simulink library "OpenFlightUtilLib"  (R2016b)
settings: Solver=VariableStepAuto  StartTime=0.0  StopTime=10.0  RelTol=1e-3
undefined symbols (not defined in the file or in its folder): SampleTime
libraries: OpenFlightUtilLib x46, simulink x7, dspmtrx3 x1
settings Model: Creator=UAVLAB  LastModifiedBy=rega0051

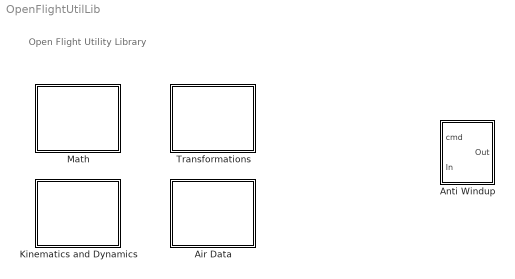
== system OpenFlightUtilLib ==
  note: Open Flight Utility Library
  Air Data : Subsystem
  Anti Windup : Subsystem  mask(Integrator Anti-Windup){MAX_DEF=0, MIN_DEF=0, gain_sign=off}
      mask prompts: MAX_DEF "Maximum surface deflection limit"; MIN_DEF "Minimum surface deflection limit"; gain_sign "Positive gains in control law"
      mask help:
      | This block uses boolean logic to eliminate integrator windup.
      | It compares the sign of the error between reference and output,
      | and the sign and position of the surface being controlled.
      mask Help:
      | See the "READ ME" block under the mask for a more thorough explanation of
      | how this block works.
  Kinematics and Dynamics : Subsystem
  Math : Subsystem
  Transformations : Subsystem

== system OpenFlightUtilLib/Air Data ==
  note: Air Data
  Angle_of_Attack : Subsystem  mask(Angle of Attack){}
      mask help: Compute the angle of attack from component velocities.
  Angle_of_Flank : Subsystem  mask(Angle of Flank){}
      mask help: Compute the angle of flank from component velocities.
  Angle_of_Sideslip : Subsystem  mask(Angle of Sideslip){}
      mask help: Compute the angle of sideslip from component velocities.
  ComponentVelocities : Subsystem  mask(Component Velocities){}
      mask help: Compute the component velocities from the True Airpeed, Angle of Attack, and Angle of Sideslip.
  ComponentVelocities_Flank : Subsystem  mask(Component Velocities){}
      mask help: Compute the component velocities from the True Airpeed, Angle of Attack, and Angle of Flank.
  DynamicPressure : Subsystem  mask(Dynamic Pressure){}
      mask help: Compute the Dynamic Pressure
  Mach : Subsystem  mask(Mach Number){}
      mask help: Compute the Mach Number
  True_Airspeed : Subsystem  mask(True Airspeed){}
      mask help: Compute the true airspeed from component velocities.
  WindAngles : Subsystem  mask(Wind Angles){}
      mask help: Compute the True Airpeed, Angle of Attack, and Angle of Sideslip from component velocities.
  WindAngles_Flank : Subsystem  mask(Wind Angles){}
      mask help: Compute the True Airpeed, Angle of Attack, and Angle of Flank from component velocities.

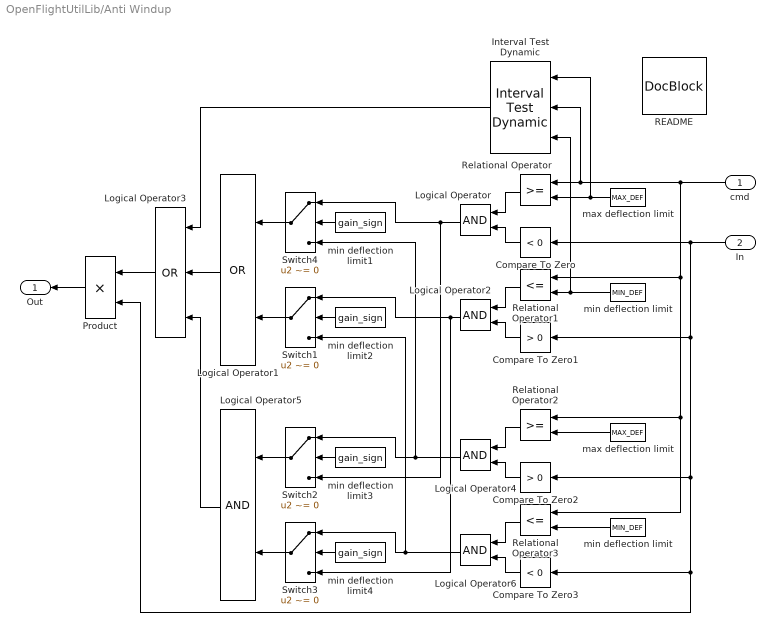
== system OpenFlightUtilLib/Anti Windup ==
  cmd : Inport
  In : Inport  Port=2
  Compare To Zero : simulink/Logic and Bit Operations/Compare To Zero  SystemSampleTime=-1  relop=<  LogicOutDataTypeMode=uint8
  Compare To Zero1 : simulink/Logic and Bit Operations/Compare To Zero  SystemSampleTime=-1  relop=>  LogicOutDataTypeMode=uint8
  Compare To Zero2 : simulink/Logic and Bit Operations/Compare To Zero  SystemSampleTime=-1  relop=>  LogicOutDataTypeMode=uint8
  Compare To Zero3 : simulink/Logic and Bit Operations/Compare To Zero  SystemSampleTime=-1  relop=<  LogicOutDataTypeMode=uint8
  Interval Test Dynamic : simulink/Logic and Bit Operations/Interval Test Dynamic  SystemSampleTime=-1  IntervalClosedRight=on  IntervalClosedLeft=on  LogicOutDataTypeMode=boolean
  Logical Operator{,2,4..6} (5 alike) : Logic  AllPortsSameDT=off  OutDataTypeStr=boolean  SampleTime=SampleTime
  Logical Operator1 : Logic  Operator=OR  AllPortsSameDT=off  OutDataTypeStr=boolean  SampleTime=SampleTime
  Logical Operator3 : Logic  Operator=OR  Inputs=3  AllPortsSameDT=off  OutDataTypeStr=boolean  SampleTime=SampleTime
  Product : Product  RndMeth=Zero
  README : simulink/Model-Wide Utilities/DocBlock  SystemSampleTime=-1  DocumentType=Text
      content=|
      | This block uses anti-windup logic to either stop or continue integrating.
      |
      | The first input signal, 'cmd', must come from the control surface command
      | that is the output of the controller. For instance, if the outputs of a PI
      | control phi tracker (with anti-windup) and a P control roll damper are
      | summed and sent to the aileron command, then the summed value must be fed
      | back into the 'cmd' input of this anti-windup block, as opposed to just the
      | output of the phi tracker.
      |
      | The second input signal, 'In', must come from the error that is being fed
      | into the control law.
      |
      | The output signal, 'Out' must feed into the error integrator block.
      |
      | For the anti-windup to work as intended, a saturation block must be placed
      | on the ouput of the control command being fed to the associated actuator.
      | If the controller is in delta coordinates, the limits in the saturation
      | block must be the actuator limits minus the trimmed control surface value.
      | For instance, for and aileron command, the limits would be:
      | Upper Limit: AC.Actuator.r_aileron.PosLim-TrimCondition.Inputs.r_aileron
      | Lower Limit: AC.Actuator.r_aileron.NegLim-TrimCondition.Inputs.r_aileron
      |
      | Depending on which surface is being controlled, the windup logic may
      | change. The default logic for this block is the following:
      |
      | For input u, saturation limits Umax and Umin, and error e,
      | If u is in bounds, do nothing
      | If u >= Umax AND e < 0, stop integrating
      | If u >= Umax AND e > 0, continue integrating
      | If u <= Umin AND e < 0, continue integrating
      | If u <= Umin AND e > 0, stop integrating
      |
      | This is the logic for a plant transfer function with a negative gain. In
      | other words, a positive input gives a negative response, which is usually
      | the case with flight dynamics. If the plant transfer function does not have
      | a negative gain, the logic will need to be reversed. In this case, the
      | inequalities on the error logic must be switched, so
      | If u is in bounds, do nothing
      | If u >= Umax AND e > 0, stop integrating
      | If u >= Umax AND e < 0, continue integrating
      | If u <= Umin AND e > 0, continue integrating
      | If u <= Umin AND e < 0, stop integrating
  Relational Operator : RelationalOperator  OutDataTypeStr=boolean  RndMeth=Nearest
  Relational Operator1 : RelationalOperator  Operator=<=  OutDataTypeStr=boolean  RndMeth=Nearest
  Relational Operator2 : RelationalOperator  OutDataTypeStr=boolean  RndMeth=Nearest
  Relational Operator3 : RelationalOperator  Operator=<=  OutDataTypeStr=boolean  RndMeth=Nearest
  Switch{1..4} (4 alike) : Switch  Criteria=u2 ~= 0  SampleTime=SampleTime
  max deflection limit : Constant  Value=MAX_DEF  SampleTime=SampleTime
  "max deflection limit " : Constant  Value=MAX_DEF  SampleTime=SampleTime
  min deflection limit : Constant  Value=MIN_DEF  SampleTime=SampleTime
  "min deflection limit " : Constant  Value=MIN_DEF  SampleTime=SampleTime
  min deflection limit{1..4} (4 alike) : Constant  Value=gain_sign  SampleTime=SampleTime
  Out : Outport
  wires:
  Logical Operator5/1 -> Logical Operator3/3
  "max deflection limit "/1 -> Relational Operator2/2
  "min deflection limit "/1 -> Relational Operator3/2
  Relational Operator3/1 -> Logical Operator6/1
  Compare To Zero3/1 -> Logical Operator6/2
  Relational Operator2/1 -> Logical Operator4/1
  Compare To Zero2/1 -> Logical Operator4/2
  Interval Test Dynamic/1 -> Logical Operator3/1
  Logical Operator1/1 -> Logical Operator3/2
  Logical Operator3/1 -> Product/1
  Product/1 -> Out/1
  min deflection limit/1 -> Interval Test Dynamic/3, Relational Operator1/2
  Relational Operator1/1 -> Logical Operator2/1
  Compare To Zero1/1 -> Logical Operator2/2
  In/1 -> Product/2, Compare To Zero3/1, Compare To Zero2/1, Compare To Zero1/1, Compare To Zero/1
  Relational Operator/1 -> Logical Operator/1
  Compare To Zero/1 -> Logical Operator/2
  cmd/1 -> Relational Operator3/1, Relational Operator2/1, Relational Operator1/1, Interval Test Dynamic/2, Relational Operator/1
  max deflection limit/1 -> Interval Test Dynamic/1, Relational Operator/2
  min deflection limit2/1 -> Switch1/2
  min deflection limit3/1 -> Switch2/2
  min deflection limit4/1 -> Switch3/2
  Switch2/1 -> Logical Operator5/1
  Switch3/1 -> Logical Operator5/2
  Switch1/1 -> Logical Operator1/2
  Switch4/1 -> Logical Operator1/1
  min deflection limit1/1 -> Switch4/2
  Logical Operator/1 -> Switch4/1, Switch2/3
  Logical Operator2/1 -> Switch1/1, Switch3/3
  Logical Operator4/1 -> Switch2/1, Switch4/3
  Logical Operator6/1 -> Switch3/1, Switch1/3

== system OpenFlightUtilLib/Kinematics and Dynamics ==
  note: Kinematics and Dynamics
  AngMomentum : Subsystem
  AngMomentumInv : Subsystem
  RelAccel : Subsystem
  RelAccelRigid : Subsystem
  RelForce : Subsystem
  RelForceRigid : Subsystem
  RelVel : Subsystem
  RelVelRigid : Subsystem
  TransMomentum : Subsystem
  TransMomentumInv : Subsystem

== system OpenFlightUtilLib/Math ==
  note: Simple Math
  CrossProduct3 : Subsystem  mask(Corss Product (3x3)){}
      mask help: Computes the cross product of two vectors of length 3.
  NormFrobenious : Subsystem
  NormL2 : Subsystem  mask(Norm L2){}
      mask help:
      | Computes the L2 Norm of a vector.
      | y = sqrt(x1^2 + x2^2 + ... + xn^2)
      mask Display: disp('||u||2');
  Psi_180_2_360 : Subsystem
  SkewSymmetric3 : Subsystem  mask(Skew Symmetric (3x3)){}
      mask help:
      | Compute the skew symmetric matrix of a vector of length 3.
      | M = [0, -V(3), V(2); V(3), 0, -V(1); -V(2), V(1), 0]
  ZeroProtect : Subsystem  mask(Zero Protection){epsilon=eps}
      mask prompts: epsilon "Epsilon value:"
      mask help:
      | Protection for divide by zero.
      | out = sign(in) * max(abs(in), eps)

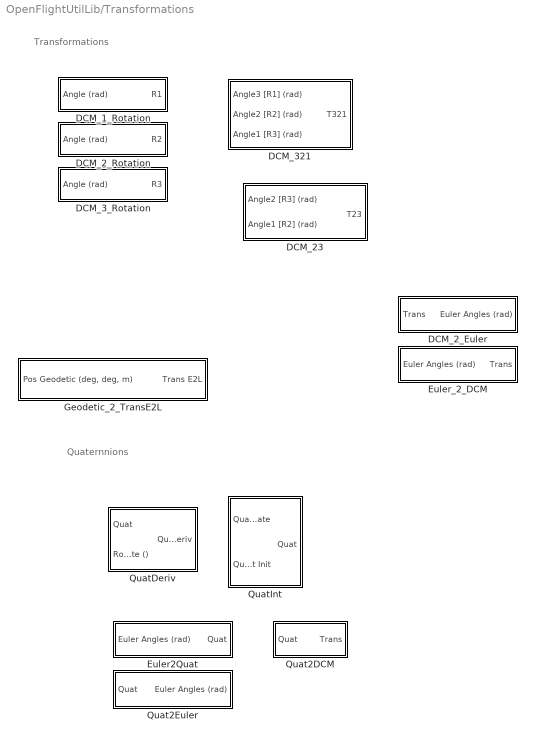
== system OpenFlightUtilLib/Transformations ==
  note: Quaternnions
  note: Transformations
  DCM_1_Rotation : Subsystem
  DCM_23 : Subsystem
  DCM_2_Euler : Subsystem
  DCM_2_Rotation : Subsystem
  DCM_321 : Subsystem
  DCM_3_Rotation : Subsystem
  Euler2Quat : Subsystem
  Euler_2_DCM : Subsystem
  Geodetic_2_TransE2L : Subsystem
  Quat2DCM : Subsystem
  Quat2Euler : Subsystem
  QuatDeriv : Subsystem
  QuatInt : Subsystem

== system OpenFlightUtilLib/Air Data/Angle_of_Attack ==
  note: alpha = atan(w / u)
  note: Convert Velocity Components to Angles of Attack
  u : Inport
  w : Inport  Port=2
  Trigonometric Function : Trigonometry  Operator=atan2
  alpha (rad) : Outport
  wires:
  Trigonometric Function/1 -> alpha (rad)/1
  u/1 -> Trigonometric Function/2
  w/1 -> Trigonometric Function/1

== system OpenFlightUtilLib/Air Data/Angle_of_Flank ==
  note: Convert Velocity Components to Angles of Flank
  note: flank = atan(v / u)
  u : Inport
  v : Inport  Port=2
  Trigonometric Function1 : Trigonometry  Operator=atan2
  flank (rad) : Outport
  wires:
  Trigonometric Function1/1 -> flank (rad)/1
  v/1 -> Trigonometric Function1/1
  u/1 -> Trigonometric Function1/2

== system OpenFlightUtilLib/Air Data/Angle_of_Sideslip ==
  note: beta = asin(v / V)
  note: Convert Velocity Components to Angles of Sideslip
  vTrue : Inport
  v : Inport  Port=2
  Product2 : Product  Inputs=*/  RndMeth=Zero
  Trigonometric Function1 : Trigonometry  Operator=asin
  ZeroProtect : OpenFlightUtilLib/Math/ZeroProtect  epsilon=eps
  beta (rad) : Outport
  wires:
  ZeroProtect/1 -> Product2/2
  Trigonometric Function1/1 -> beta (rad)/1
  Product2/1 -> Trigonometric Function1/1
  v/1 -> Product2/1
  vTrue/1 -> ZeroProtect/1

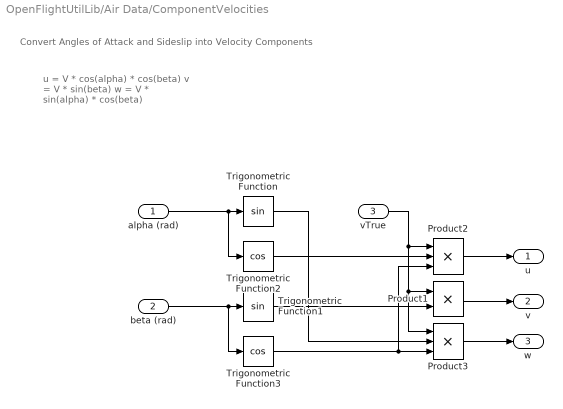
== system OpenFlightUtilLib/Air Data/ComponentVelocities ==
  note: u = V * cos(alpha) * cos(beta)
      | v = V * sin(beta)
      | w = V * sin(alpha) * cos(beta)
  note: Convert Angles of Attack and Sideslip into Velocity Components
  alpha (rad) : Inport
  beta (rad) : Inport  Port=2
  vTrue : Inport  Port=3
  Product1 : Product  Inputs=**  RndMeth=Zero
  Product2 : Product  Inputs=***  RndMeth=Zero
  Product3 : Product  Inputs=***  RndMeth=Zero
  Trigonometric Function : Trigonometry
  Trigonometric Function1 : Trigonometry
  Trigonometric Function2 : Trigonometry  Operator=cos
  Trigonometric Function3 : Trigonometry  Operator=cos
  u : Outport
  v : Outport  Port=2
  w : Outport  Port=3
  wires:
  Product3/1 -> w/1
  Product1/1 -> v/1
  beta (rad)/1 -> Trigonometric Function1/1, Trigonometric Function3/1
  alpha (rad)/1 -> Trigonometric Function/1, Trigonometric Function2/1
  Product2/1 -> u/1
  Trigonometric Function1/1 -> Product1/2
  Trigonometric Function/1 -> Product3/2
  vTrue/1 -> Product2/1, Product1/1, Product3/1
  Trigonometric Function2/1 -> Product2/2
  Trigonometric Function3/1 -> Product2/3, Product3/3

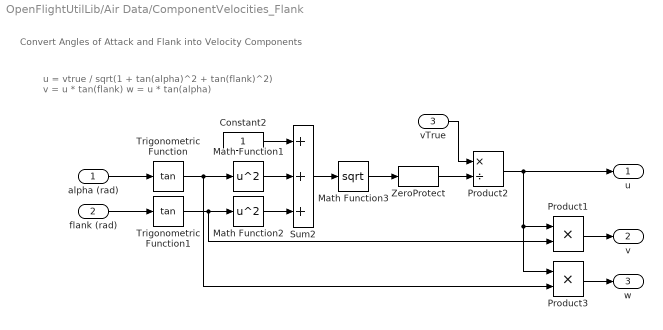
== system OpenFlightUtilLib/Air Data/ComponentVelocities_Flank ==
  note: Convert Angles of Attack and Flank into Velocity Components
  note: u = vtrue / sqrt(1 + tan(alpha)^2 + tan(flank)^2)
      | v = u * tan(flank)
      | w = u * tan(alpha)
  alpha (rad) : Inport
  flank (rad) : Inport  Port=2
  vTrue : Inport  Port=3
  Constant2 : Constant
  Math Function1 : Math  Operator=square  SaturateOnIntegerOverflow=on
  Math Function2 : Math  Operator=square  SaturateOnIntegerOverflow=on
  Math Function3 : Math  Operator=sqrt  SaturateOnIntegerOverflow=on
  Product1 : Product  Inputs=**  RndMeth=Zero
  Product2 : Product  Inputs=*/  RndMeth=Zero
  Product3 : Product  Inputs=**  RndMeth=Zero
  Sum2 : Sum  Inputs=+++
  Trigonometric Function : Trigonometry  Operator=tan
  Trigonometric Function1 : Trigonometry  Operator=tan
  ZeroProtect : OpenFlightUtilLib/Math/ZeroProtect  epsilon=eps
  u : Outport
  v : Outport  Port=2
  w : Outport  Port=3
  wires:
  vTrue/1 -> Product2/1
  Sum2/1 -> Math Function3/1
  Math Function3/1 -> ZeroProtect/1
  Trigonometric Function/1 -> Math Function1/1, Product3/2
  Trigonometric Function1/1 -> Math Function2/1, Product1/2
  Product2/1 -> u/1, Product1/1, Product3/1
  alpha (rad)/1 -> Trigonometric Function/1
  flank (rad)/1 -> Trigonometric Function1/1
  Product1/1 -> v/1
  Product3/1 -> w/1
  Constant2/1 -> Sum2/1
  Math Function1/1 -> Sum2/2
  Math Function2/1 -> Sum2/3
  ZeroProtect/1 -> Product2/2

== system OpenFlightUtilLib/Air Data/DynamicPressure ==
  note: qBar = 0.5 * rho * V^2
  note: Compute Dynamic Pressure
  vTrue : Inport
  density : Inport  Port=2
  Gain : Gain  Gain=1/2
  Math Function : Math  Operator=square  SaturateOnIntegerOverflow=on
  Product2 : Product  Inputs=**  RndMeth=Zero
  qBar : Outport
  wires:
  density/1 -> Product2/2
  vTrue/1 -> Math Function/1
  Product2/1 -> Gain/1
  Gain/1 -> qBar/1
  Math Function/1 -> Product2/1

== system OpenFlightUtilLib/Air Data/Mach ==
  note: Compute Mach Number
  note: mach = vTrue / vSound
  vTrue : Inport
  vSound : Inport  Port=2
  Product2 : Product  Inputs=*/  RndMeth=Zero
  ZeroProtect : OpenFlightUtilLib/Math/ZeroProtect  epsilon=eps
  mach : Outport
  wires:
  Product2/1 -> mach/1
  vSound/1 -> ZeroProtect/1
  vTrue/1 -> Product2/1
  ZeroProtect/1 -> Product2/2

== system OpenFlightUtilLib/Air Data/True_Airspeed ==
  note: V = sqrt(u^2 + v^2 + w^2)
  note: Convert Velocity Components to True Airspeed
  u : Inport
  v : Inport  Port=2
  w : Inport  Port=3
  Mux : Mux  Inputs=3
  NormL2 : OpenFlightUtilLib/Math/NormL2
  vTrue : Outport
  wires:
  Mux/1 -> NormL2/1
  u/1 -> Mux/1
  v/1 -> Mux/2
  w/1 -> Mux/3
  NormL2/1 -> vTrue/1

== system OpenFlightUtilLib/Air Data/WindAngles ==
  note: Convert Velocity Components to True Airspeed, Angles of Attack, and Sideslip
  u : Inport
  v : Inport  Port=2
  w : Inport  Port=3
  Angle_of_Attack : OpenFlightUtilLib/Air Data/Angle_of_Attack
  Angle_of_Sideslip1 : OpenFlightUtilLib/Air Data/Angle_of_Sideslip
  True_Airspeed : OpenFlightUtilLib/Air Data/True_Airspeed
  vTrue : Outport
  alpha (rad) : Outport  Port=2
  beta (rad) : Outport  Port=3
  wires:
  True_Airspeed/1 -> Angle_of_Sideslip1/1, vTrue/1
  Angle_of_Attack/1 -> alpha (rad)/1
  Angle_of_Sideslip1/1 -> beta (rad)/1
  u/1 -> True_Airspeed/1, Angle_of_Attack/1
  v/1 -> True_Airspeed/2, Angle_of_Sideslip1/2
  w/1 -> True_Airspeed/3, Angle_of_Attack/2

== system OpenFlightUtilLib/Air Data/WindAngles_Flank ==
  note: V = sqrt(u^2 + v^2 + w^2)
      | alpha = atan(w / u)
      | flank = atan(v / u)
  note: Convert Velocity Components to Angles of Attack and Flank
  u : Inport
  v : Inport  Port=2
  w : Inport  Port=3
  Angle_of_Attack : OpenFlightUtilLib/Air Data/Angle_of_Attack
  Angle_of_Flank : OpenFlightUtilLib/Air Data/Angle_of_Flank
  True_Airspeed : OpenFlightUtilLib/Air Data/True_Airspeed
  vTrue : Outport
  alpha (rad) : Outport  Port=2
  flank (rad) : Outport  Port=3
  wires:
  u/1 -> True_Airspeed/1, Angle_of_Flank/1, Angle_of_Attack/1
  v/1 -> Angle_of_Flank/2, True_Airspeed/2
  w/1 -> Angle_of_Attack/2, True_Airspeed/3
  True_Airspeed/1 -> vTrue/1
  Angle_of_Attack/1 -> alpha (rad)/1
  Angle_of_Flank/1 -> flank (rad)/1

== system OpenFlightUtilLib/Kinematics and Dynamics/AngMomentum ==
  note: Rigid Body Conservation of Angular Momentum
  note: M = Idot*w + I*wdot + w X (I*w)
      | wdot = inv(I)*(M - Idot*w - w X (I*w))
  w : Inport
  I : Inport  Port=2
  IDot : Inport  Port=3
  wDot : Inport  Port=4
  Cross_Product_(3X3) : OpenFlightUtilLib/Math/CrossProduct3
  Product1 : Product  Inputs=**  Multiplication=Matrix(*)  SaturateOnIntegerOverflow=on  OutDataTypeStr=Inherit: Same as first input
  Product2 : Product  Multiplication=Matrix(*)  SaturateOnIntegerOverflow=on  OutDataTypeStr=Inherit: Same as first input
  Product3 : Product  Multiplication=Matrix(*)  SaturateOnIntegerOverflow=on  OutDataTypeStr=Inherit: Same as first input
  Reshape : Reshape  OutputDimensionality=Customize  OutputDimensions=[3,1]
  Sum1 : Sum  Inputs=+++  SaturateOnIntegerOverflow=on
  M : Outport
  wires:
  Sum1/1 -> M/1
  Product1/1 -> Sum1/3
  Reshape/1 -> Cross_Product_(3X3)/1, Product2/2, Product3/2
  wDot/1 -> Product1/2
  I/1 -> Product1/1, Product2/1
  w/1 -> Reshape/1
  Product2/1 -> Cross_Product_(3X3)/2
  IDot/1 -> Product3/1
  Product3/1 -> Sum1/1
  Cross_Product_(3X3)/1 -> Sum1/2

== system OpenFlightUtilLib/Kinematics and Dynamics/AngMomentumInv ==
  note: Rigid Body Conservation of Angular Momentum - Inverse
  note: M = Idot*w + I*wdot + w X (I*w)
      | wdot = inv(I)*(M - Idot*w - w X (I*w))
  w : Inport
  I : Inport  Port=2
  IDot : Inport  Port=3
  M : Inport  Port=4
  CrossProduct3 : OpenFlightUtilLib/Math/CrossProduct3
  Product1 : Product  Inputs=/*  Multiplication=Matrix(*)  SaturateOnIntegerOverflow=on  OutDataTypeStr=Inherit: Same as first input
  Product2 : Product  Multiplication=Matrix(*)  SaturateOnIntegerOverflow=on  OutDataTypeStr=Inherit: Same as first input
  Product3 : Product  Multiplication=Matrix(*)  SaturateOnIntegerOverflow=on  OutDataTypeStr=Inherit: Same as first input
  Reshape : Reshape  OutputDimensionality=Customize  OutputDimensions=[3,1]
  Sum1 : Sum  Inputs=--+  SaturateOnIntegerOverflow=on
  ZeroProtect : OpenFlightUtilLib/Math/ZeroProtect  epsilon=eps
  wDot : Outport
  wires:
  ZeroProtect/1 -> Product1/1
  M/1 -> Sum1/3
  Sum1/1 -> Product1/2
  CrossProduct3/1 -> Sum1/2
  Reshape/1 -> CrossProduct3/1, Product3/2, Product2/2
  Product1/1 -> wDot/1
  Product3/1 -> Sum1/1
  IDot/1 -> Product3/1
  Product2/1 -> CrossProduct3/2
  w/1 -> Reshape/1
  I/1 -> ZeroProtect/1, Product2/1

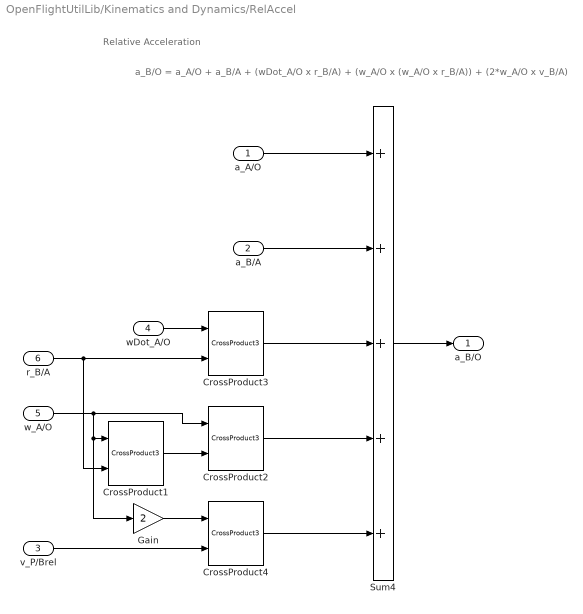
== system OpenFlightUtilLib/Kinematics and Dynamics/RelAccel ==
  note: a_B/O = a_A/O + a_B/A + (wDot_A/O x r_B/A) + (w_A/O x (w_A/O x r_B/A)) + (2*w_A/O x v_B/A)
  note: Relative Acceleration
  a_A/O : Inport
  a_B/A : Inport  Port=2
  v_P/Brel : Inport  Port=3
  wDot_A/O : Inport  Port=4
  w_A/O : Inport  Port=5
  r_B/A : Inport  Port=6
  CrossProduct{1..4} (4 alike) : OpenFlightUtilLib/Math/CrossProduct3
  Gain : Gain  Gain=2
  Sum4 : Sum  Inputs=+++++
  a_B/O : Outport
  wires:
  CrossProduct1/1 -> CrossProduct2/2
  r_B/A/1 -> CrossProduct1/2, CrossProduct3/2
  wDot_A/O/1 -> CrossProduct3/1
  Sum4/1 -> a_B/O/1
  v_P/Brel/1 -> CrossProduct4/2
  Gain/1 -> CrossProduct4/1
  w_A/O/1 -> CrossProduct2/1, CrossProduct1/1, Gain/1
  a_A/O/1 -> Sum4/1
  a_B/A/1 -> Sum4/2
  CrossProduct3/1 -> Sum4/3
  CrossProduct2/1 -> Sum4/4
  CrossProduct4/1 -> Sum4/5

== system OpenFlightUtilLib/Kinematics and Dynamics/RelAccelRigid ==
  note: Relative Acceleration - Rigid Body (A and B are on a rigid body)
  note: a_B/O = a_A/O + (wDot_A/O x r_B/A) + (w_A/O x (w_A/O x r_B/A))
  a_A/O : Inport
  wDot_A/O : Inport  Port=2
  w_A/O : Inport  Port=3
  r_B/A : Inport  Port=4
  CrossProduct1 : OpenFlightUtilLib/Math/CrossProduct3
  CrossProduct2 : OpenFlightUtilLib/Math/CrossProduct3
  CrossProduct3 : OpenFlightUtilLib/Math/CrossProduct3
  Sum4 : Sum  Inputs=+++
  a_B/O : Outport
  wires:
  CrossProduct2/1 -> Sum4/3
  CrossProduct3/1 -> Sum4/2
  a_A/O/1 -> Sum4/1
  w_A/O/1 -> CrossProduct1/1, CrossProduct2/1
  Sum4/1 -> a_B/O/1
  wDot_A/O/1 -> CrossProduct3/1
  r_B/A/1 -> CrossProduct3/2, CrossProduct1/2
  CrossProduct1/1 -> CrossProduct2/2

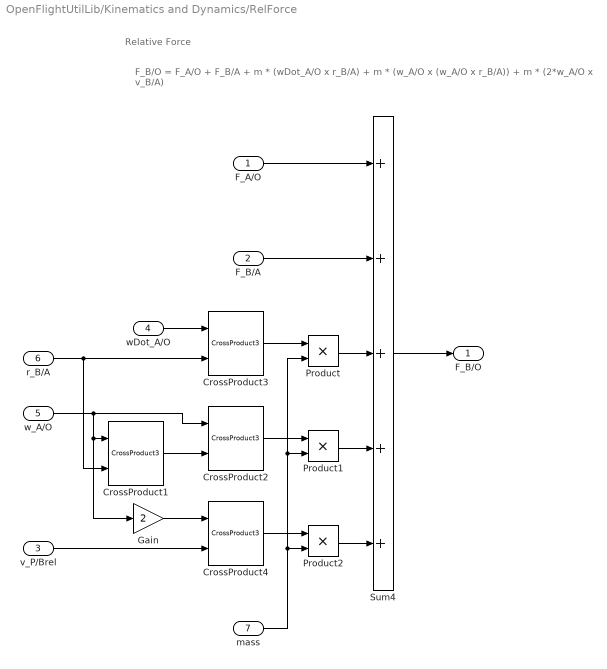
== system OpenFlightUtilLib/Kinematics and Dynamics/RelForce ==
  note: Relative Force
  note: F_B/O = F_A/O + F_B/A + m * (wDot_A/O x r_B/A) + m * (w_A/O x (w_A/O x r_B/A)) + m * (2*w_A/O x v_B/A)
  F_A/O : Inport
  F_B/A : Inport  Port=2
  v_P/Brel : Inport  Port=3
  wDot_A/O : Inport  Port=4
  w_A/O : Inport  Port=5
  r_B/A : Inport  Port=6
  mass : Inport  Port=7
  CrossProduct{1..4} (4 alike) : OpenFlightUtilLib/Math/CrossProduct3
  Gain : Gain  Gain=2
  Product : Product
  Product1 : Product
  Product2 : Product
  Sum4 : Sum  Inputs=+++++
  F_B/O : Outport
  wires:
  CrossProduct3/1 -> Product/1
  F_B/A/1 -> Sum4/2
  F_A/O/1 -> Sum4/1
  w_A/O/1 -> Gain/1, CrossProduct1/1, CrossProduct2/1
  Gain/1 -> CrossProduct4/1
  v_P/Brel/1 -> CrossProduct4/2
  Sum4/1 -> F_B/O/1
  wDot_A/O/1 -> CrossProduct3/1
  r_B/A/1 -> CrossProduct3/2, CrossProduct1/2
  CrossProduct1/1 -> CrossProduct2/2
  Product/1 -> Sum4/3
  CrossProduct2/1 -> Product1/1
  Product1/1 -> Sum4/4
  Product2/1 -> Sum4/5
  CrossProduct4/1 -> Product2/1
  mass/1 -> Product/2, Product1/2, Product2/2

== system OpenFlightUtilLib/Kinematics and Dynamics/RelForceRigid ==
  note: F_B/O = F_A/O + m * (wDot_A/O x r_B/A) + m * (w_A/O x (w_A/O x r_B/A))
  note: Relative Force - Rigid Body (A and B are on a rigid body)
  F_A/O : Inport
  wDot_A/O : Inport  Port=2
  w_A/O : Inport  Port=3
  r_B/A : Inport  Port=4
  mass : Inport  Port=5
  CrossProduct1 : OpenFlightUtilLib/Math/CrossProduct3
  CrossProduct2 : OpenFlightUtilLib/Math/CrossProduct3
  CrossProduct3 : OpenFlightUtilLib/Math/CrossProduct3
  Product : Product
  Product1 : Product
  Sum4 : Sum  Inputs=+++
  F_B/O : Outport
  wires:
  CrossProduct1/1 -> CrossProduct2/2
  r_B/A/1 -> CrossProduct1/2, CrossProduct3/2
  wDot_A/O/1 -> CrossProduct3/1
  Sum4/1 -> F_B/O/1
  w_A/O/1 -> CrossProduct2/1, CrossProduct1/1
  F_A/O/1 -> Sum4/1
  CrossProduct3/1 -> Product/1
  Product/1 -> Sum4/2
  Product1/1 -> Sum4/3
  CrossProduct2/1 -> Product1/1
  mass/1 -> Product1/2, Product/2

== system OpenFlightUtilLib/Kinematics and Dynamics/RelVel ==
  note: Relative Velocity
  note: v_B/O = v_A/O + v_B/A + (w_A/O x r_B/A)
  v_A/O : Inport
  v_B/A : Inport  Port=2
  w_A/O : Inport  Port=3
  r_B/A : Inport  Port=4
  CrossProduct3 : OpenFlightUtilLib/Math/CrossProduct3
  Sum1 : Sum  Inputs=+++
  v_B/O : Outport
  wires:
  v_A/O/1 -> Sum1/1
  v_B/A/1 -> Sum1/2
  CrossProduct3/1 -> Sum1/3
  Sum1/1 -> v_B/O/1
  w_A/O/1 -> CrossProduct3/1
  r_B/A/1 -> CrossProduct3/2

== system OpenFlightUtilLib/Kinematics and Dynamics/RelVelRigid ==
  note: v_B/O = v_A/O + (w_A/O x r_B/A)
  note: Relative Velocity - Rigid Body (A and B are on a rigid body)
  v_A/O : Inport
  w_A/O : Inport  Port=2
  r_B/A : Inport  Port=3
  CrossProduct3 : OpenFlightUtilLib/Math/CrossProduct3
  Sum1 : Sum
  v_B/O : Outport
  wires:
  r_B/A/1 -> CrossProduct3/2
  w_A/O/1 -> CrossProduct3/1
  Sum1/1 -> v_B/O/1
  CrossProduct3/1 -> Sum1/2
  v_A/O/1 -> Sum1/1

== system OpenFlightUtilLib/Kinematics and Dynamics/TransMomentum ==
  note: Rigid Body Conservation of Momentum
  note: F = mdot*v + m*vdot + w X (m*v)
      | vdot = (1/m)*(F - mdot*v - w X (m*v))
  v : Inport
  m : Inport  Port=2
  vDot : Inport  Port=3
  mDot : Inport  Port=4
  w : Inport  Port=5
  CrossProduct3 : OpenFlightUtilLib/Math/CrossProduct3
  Product1 : Product  Inputs=**  SaturateOnIntegerOverflow=on  OutDataTypeStr=Inherit: Same as first input
  Product2 : Product  SaturateOnIntegerOverflow=on  OutDataTypeStr=Inherit: Same as first input
  Product3 : Product  SaturateOnIntegerOverflow=on  OutDataTypeStr=Inherit: Same as first input
  Reshape : Reshape  OutputDimensionality=Customize  OutputDimensions=[3,1]
  Reshape1 : Reshape  OutputDimensionality=Customize  OutputDimensions=[3,1]
  Sum1 : Sum  Inputs=+++  SaturateOnIntegerOverflow=on
  F : Outport
  wires:
  Reshape1/1 -> CrossProduct3/1
  w/1 -> Reshape1/1
  CrossProduct3/1 -> Sum1/2
  Product3/1 -> Sum1/1
  mDot/1 -> Product3/1
  Product2/1 -> CrossProduct3/2
  v/1 -> Reshape/1
  m/1 -> Product2/1, Product1/1
  vDot/1 -> Product1/2
  Reshape/1 -> Product3/2, Product2/2
  Product1/1 -> Sum1/3
  Sum1/1 -> F/1

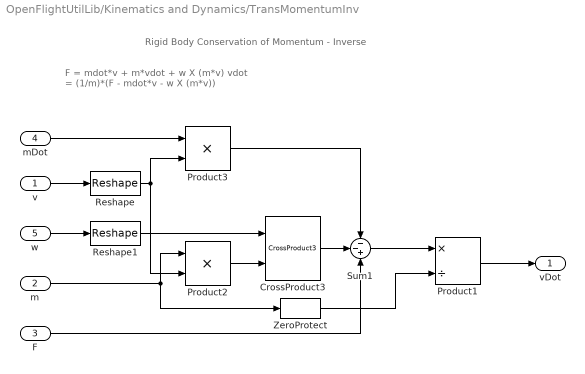
== system OpenFlightUtilLib/Kinematics and Dynamics/TransMomentumInv ==
  note: Rigid Body Conservation of Momentum - Inverse
  note: F = mdot*v + m*vdot + w X (m*v)
      | vdot = (1/m)*(F - mdot*v - w X (m*v))
  v : Inport
  m : Inport  Port=2
  F : Inport  Port=3
  mDot : Inport  Port=4
  w : Inport  Port=5
  CrossProduct3 : OpenFlightUtilLib/Math/CrossProduct3
  Product1 : Product  Inputs=*/  SaturateOnIntegerOverflow=on  OutDataTypeStr=Inherit: Same as first input
  Product2 : Product  SaturateOnIntegerOverflow=on  OutDataTypeStr=Inherit: Same as first input
  Product3 : Product  SaturateOnIntegerOverflow=on  OutDataTypeStr=Inherit: Same as first input
  Reshape : Reshape  OutputDimensionality=Customize  OutputDimensions=[3,1]
  Reshape1 : Reshape  OutputDimensionality=Customize  OutputDimensions=[3,1]
  Sum1 : Sum  Inputs=--+  SaturateOnIntegerOverflow=on
  ZeroProtect : OpenFlightUtilLib/Math/ZeroProtect  epsilon=eps
  vDot : Outport
  wires:
  ZeroProtect/1 -> Product1/2
  Product1/1 -> vDot/1
  Sum1/1 -> Product1/1
  F/1 -> Sum1/3
  Reshape/1 -> Product2/2, Product3/2
  m/1 -> ZeroProtect/1, Product2/1
  v/1 -> Reshape/1
  Product2/1 -> CrossProduct3/2
  mDot/1 -> Product3/1
  Product3/1 -> Sum1/1
  CrossProduct3/1 -> Sum1/2
  w/1 -> Reshape1/1
  Reshape1/1 -> CrossProduct3/1

== system OpenFlightUtilLib/Math/CrossProduct3 ==
  In1 : Inport
  In2 : Inport  Port=2
  Product : Product  SaturateOnIntegerOverflow=on  InputSameDT=on  OutDataTypeStr=Inherit: Same as first input
  Product1 : Product  SaturateOnIntegerOverflow=on  InputSameDT=on  OutDataTypeStr=Inherit: Same as first input
  Selector : Selector  InputPortWidth=3  IndexOptions=Index vector (dialog)  Indices=[2 3 1]  OutputSizes=1
  Selector1 : Selector  InputPortWidth=3  IndexOptions=Index vector (dialog)  Indices=[3 1 2]  OutputSizes=1
  Selector2 : Selector  InputPortWidth=3  IndexOptions=Index vector (dialog)  Indices=[2 3 1]  OutputSizes=1
  Selector3 : Selector  InputPortWidth=3  IndexOptions=Index vector (dialog)  Indices=[3 1 2]  OutputSizes=1
  Sum : Sum  Inputs=+|-  SaturateOnIntegerOverflow=on  InputSameDT=on  OutDataTypeStr=Inherit: Same as first input
  Out : Outport
  wires:
  Selector3/1 -> Product1/1
  Selector2/1 -> Product1/2
  Product1/1 -> Sum/2
  Selector1/1 -> Product/2
  Product/1 -> Sum/1
  In1/1 -> Selector3/1, Selector/1
  Selector/1 -> Product/1
  In2/1 -> Selector2/1, Selector1/1
  Sum/1 -> Out/1

== system OpenFlightUtilLib/Math/NormFrobenious ==
  note: sqrt(sum(diag(X'*X)))
  Matrix : Inport
  Extract Diagonal : dspmtrx3/Extract Diagonal
  Math Function : Math  Operator=transpose  SaturateOnIntegerOverflow=on
  Math Function1 : Math  Operator=sqrt  SaturateOnIntegerOverflow=on
  Product : Product  Multiplication=Matrix(*)  RndMeth=Zero
  Sum of Elements : Sum  Inputs=+
  Norm : Outport
  wires:
  Product/1 -> Extract Diagonal/1
  Extract Diagonal/1 -> Sum of Elements/1
  Sum of Elements/1 -> Math Function1/1
  Math Function1/1 -> Norm/1
  Matrix/1 -> Product/2, Math Function/1
  Math Function/1 -> Product/1

== system OpenFlightUtilLib/Math/NormL2 ==
  note: y = sqrt(x1^2 + x2^2 + ... + xn^2)
  note: L2 Norm of a Vector
  Vector : Inport
  Dot Product : DotProduct  InputSameDT=on  OutDataTypeStr=Inherit: Inherit via internal rule
  Math Function : Math  Operator=sqrt  SaturateOnIntegerOverflow=on
  Norm : Outport
  wires:
  Dot Product/1 -> Math Function/1
  Math Function/1 -> Norm/1
  Vector/1 -> Dot Product/1, Dot Product/2

== system OpenFlightUtilLib/Math/Psi_180_2_360 ==
  note: Convert Psi180 [-180, 180] to Psi360 [0, 360]
  Psi180 (deg) : Inport
  Constant : Constant  Value=360
  Math Function : Math  Operator=mod  SaturateOnIntegerOverflow=on
  Psi360 (deg) : Outport
  wires:
  Math Function/1 -> Psi360 (deg)/1
  Constant/1 -> Math Function/2
  Psi180 (deg)/1 -> Math Function/1

== system OpenFlightUtilLib/Math/SkewSymmetric3 ==
  note: Convert Vector to Skew Symmetric Matrix
  note: M = [0, -V(3), V(2); V(3), 0, -V(1); -V(2), V(1), 0]
  Vector : Inport
  Constant2 : Constant  Value=0
  Demux : Demux  Outputs=3
  Gain : Gain  Gain=-1
  Gain1 : Gain  Gain=-1
  Gain2 : Gain  Gain=-1
  Mux : Mux  Inputs=9
  Reshape : Reshape  OutputDimensionality=Customize  OutputDimensions=[3,3]
  Matirx : Outport
  wires:
  Gain2/1 -> Mux/8
  Gain1/1 -> Mux/4
  Gain/1 -> Mux/3
  Demux/2 -> Gain/1, Mux/7
  Demux/1 -> Gain2/1, Mux/6
  Demux/3 -> Gain1/1, Mux/2
  Reshape/1 -> Matirx/1
  Constant2/1 -> Mux/1, Mux/9, Mux/5
  Mux/1 -> Reshape/1
  Vector/1 -> Demux/1

== system OpenFlightUtilLib/Math/ZeroProtect ==
  note: Zero Protection
  note: out = sign(in) * max(abs(in), eps)
  In : Inport
  Abs : Abs
  Compare To Zero : simulink/Logic and Bit Operations/Compare To Zero  relop=>=  OutDataTypeStr=boolean  ZeroCross=off
  Constant : Constant  Value=epsilon
  Gain : Gain  Gain=-1
  Relational Operator : RelationalOperator  OutDataTypeStr=boolean  RndMeth=Nearest
  Switch : Switch  Criteria=u2 ~= 0
  Switch1 : Switch  Criteria=u2 ~= 0
  Out : Outport
  wires:
  In/1 -> Compare To Zero/1, Abs/1, Switch1/3
  Compare To Zero/1 -> Switch/2
  Gain/1 -> Switch/3
  Constant/1 -> Switch/1, Gain/1, Relational Operator/1
  Abs/1 -> Relational Operator/2
  Relational Operator/1 -> Switch1/2
  Switch/1 -> Switch1/1
  Switch1/1 -> Out/1

== system OpenFlightUtilLib/Transformations/DCM_1_Rotation ==
  note: R = [1 0 0; 0 cos sin; 0 -sin cos]
  note: Direction Cosine Matrix - 1-rotation
  Angle (rad) : Inport
  Constant1 : Constant
  Constant2 : Constant  Value=0
  Gain : Gain  Gain=-1
  Mux : Mux  Inputs=9
  Reshape : Reshape  OutputDimensionality=Customize  OutputDimensions=[3,3]
  Trigonometric Function : Trigonometry
  Trigonometric Function1 : Trigonometry  Operator=cos
  R1 : Outport
  wires:
  Gain/1 -> Mux/6
  Reshape/1 -> R1/1
  Mux/1 -> Reshape/1
  Trigonometric Function/1 -> Mux/8, Gain/1
  Trigonometric Function1/1 -> Mux/9, Mux/5
  Angle (rad)/1 -> Trigonometric Function1/1, Trigonometric Function/1
  Constant2/1 -> Mux/2, Mux/3, Mux/7, Mux/4
  Constant1/1 -> Mux/1

== system OpenFlightUtilLib/Transformations/DCM_23 ==
  note: T23 = R3 * R2
  note: Direction Cosine Matrix - 23-rotation
  Angle2 [R3] (rad) : Inport
  Angle1 [R2] (rad) : Inport  Port=2
  DCM_2_Rotation : OpenFlightUtilLib/Transformations/DCM_2_Rotation
  DCM_3_Rotation : OpenFlightUtilLib/Transformations/DCM_3_Rotation
  Product : Product  Multiplication=Matrix(*)  RndMeth=Zero
  T23 : Outport
  wires:
  Product/1 -> T23/1
  DCM_2_Rotation/1 -> Product/2
  DCM_3_Rotation/1 -> Product/1
  Angle2 [R3] (rad)/1 -> DCM_3_Rotation/1
  Angle1 [R2] (rad)/1 -> DCM_2_Rotation/1

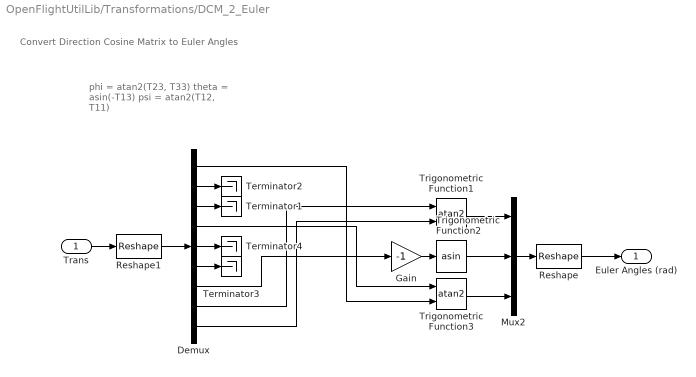
== system OpenFlightUtilLib/Transformations/DCM_2_Euler ==
  note: phi = atan2(T23, T33)
      | theta = asin(-T13)
      | psi = atan2(T12, T11)
  note: Convert Direction Cosine Matrix to Euler Angles
  Trans : Inport
  Demux : Demux  Outputs=9
  Gain : Gain  Gain=-1
  Mux2 : Mux  Inputs=3
  Reshape : Reshape  OutputDimensionality=Customize  OutputDimensions=[3,1]
  Reshape1 : Reshape  OutputDimensionality=Customize  OutputDimensions=[9,1]
  Terminator{1..4} (4 alike) : Terminator
  Trigonometric Function1 : Trigonometry  Operator=atan2
  Trigonometric Function2 : Trigonometry  Operator=asin
  Trigonometric Function3 : Trigonometry  Operator=atan2
  Euler Angles (rad) : Outport
  wires:
  Demux/6 -> Terminator3/1
  Demux/5 -> Terminator4/1
  Demux/3 -> Terminator1/1
  Demux/2 -> Terminator2/1
  Demux/1 -> Trigonometric Function3/2
  Demux/4 -> Trigonometric Function3/1
  Demux/9 -> Trigonometric Function1/2
  Demux/8 -> Trigonometric Function1/1
  Demux/7 -> Gain/1
  Gain/1 -> Trigonometric Function2/1
  Reshape1/1 -> Demux/1
  Reshape/1 -> Euler Angles (rad)/1
  Mux2/1 -> Reshape/1
  Trigonometric Function3/1 -> Mux2/3
  Trigonometric Function2/1 -> Mux2/2
  Trigonometric Function1/1 -> Mux2/1
  Trans/1 -> Reshape1/1

== system OpenFlightUtilLib/Transformations/DCM_2_Rotation ==
  note: Direction Cosine Matrix - 2-rotation
  note: R2 = [cos 0 -sin; 0 1 0; sin 0 cos]
  Angle (rad) : Inport
  Constant1 : Constant
  Constant2 : Constant  Value=0
  Gain : Gain  Gain=-1
  Mux : Mux  Inputs=9
  Reshape : Reshape  OutputDimensionality=Customize  OutputDimensions=[3,3]
  Trigonometric Function : Trigonometry
  Trigonometric Function1 : Trigonometry  Operator=cos
  R2 : Outport
  wires:
  Constant2/1 -> Mux/6, Mux/8, Mux/4, Mux/2
  Constant1/1 -> Mux/5
  Reshape/1 -> R2/1
  Angle (rad)/1 -> Trigonometric Function/1, Trigonometric Function1/1
  Trigonometric Function/1 -> Mux/3, Gain/1
  Trigonometric Function1/1 -> Mux/1, Mux/9
  Gain/1 -> Mux/7
  Mux/1 -> Reshape/1

== system OpenFlightUtilLib/Transformations/DCM_321 ==
  note: Direction Cosine Matrix - 321-rotation
  note: T321 = R1 * (R2 * R3)
  Angle3 [R1] (rad) : Inport
  Angle2 [R2] (rad) : Inport  Port=2
  Angle1 [R3] (rad) : Inport  Port=3
  DCM_1_Rotation : OpenFlightUtilLib/Transformations/DCM_1_Rotation
  DCM_2_Rotation : OpenFlightUtilLib/Transformations/DCM_2_Rotation
  DCM_3_Rotation : OpenFlightUtilLib/Transformations/DCM_3_Rotation
  Product : Product  Multiplication=Matrix(*)  RndMeth=Zero
  Product1 : Product  Multiplication=Matrix(*)  RndMeth=Zero
  T321 : Outport
  wires:
  Angle1 [R3] (rad)/1 -> DCM_3_Rotation/1
  Angle2 [R2] (rad)/1 -> DCM_2_Rotation/1
  DCM_3_Rotation/1 -> Product/2
  DCM_2_Rotation/1 -> Product/1
  Product/1 -> Product1/2
  DCM_1_Rotation/1 -> Product1/1
  Angle3 [R1] (rad)/1 -> DCM_1_Rotation/1
  Product1/1 -> T321/1

== system OpenFlightUtilLib/Transformations/DCM_3_Rotation ==
  note: R3 = [cos sin 0; -sin cos 0; 0 0 1]
  note: Direction Cosine Matrix - 3-rotation
  Angle (rad) : Inport
  Constant1 : Constant
  Constant2 : Constant  Value=0
  Gain : Gain  Gain=-1
  Mux : Mux  Inputs=9
  Reshape : Reshape  OutputDimensionality=Customize  OutputDimensions=[3,3]
  Trigonometric Function : Trigonometry
  Trigonometric Function1 : Trigonometry  Operator=cos
  R3 : Outport
  wires:
  Gain/1 -> Mux/2
  Reshape/1 -> R3/1
  Mux/1 -> Reshape/1
  Trigonometric Function1/1 -> Mux/1, Mux/5
  Constant2/1 -> Mux/3, Mux/6, Mux/7, Mux/8
  Constant1/1 -> Mux/9
  Trigonometric Function/1 -> Gain/1, Mux/4
  Angle (rad)/1 -> Trigonometric Function1/1, Trigonometric Function/1

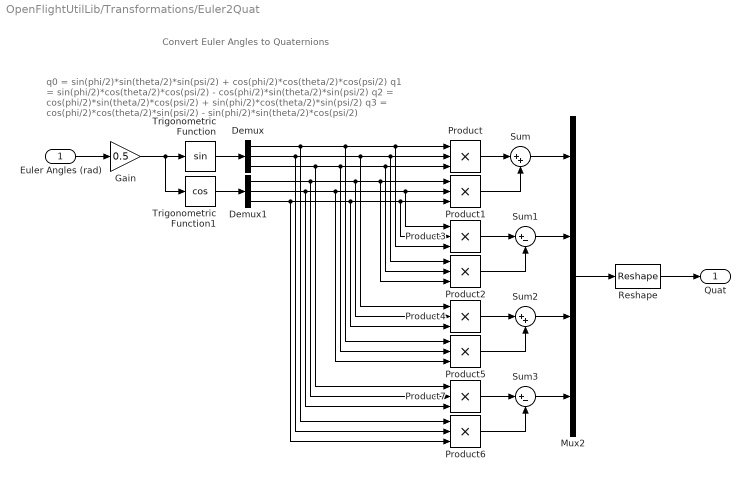
== system OpenFlightUtilLib/Transformations/Euler2Quat ==
  note: q0 = sin(phi/2)*sin(theta/2)*sin(psi/2) + cos(phi/2)*cos(theta/2)*cos(psi/2)
      | q1 = sin(phi/2)*cos(theta/2)*cos(psi/2) - cos(phi/2)*sin(theta/2)*sin(psi/2)
      | q2 = cos(phi/2)*sin(theta/2)*cos(psi/2) + sin(phi/2)*cos(theta/2)*sin(psi/2)
      | q3 = cos(phi/2)*cos(theta/2)*sin(psi/2) - sin(phi/2)*sin(theta/2)*cos(psi/2)
  note: Convert Euler Angles to Quaternions
  Euler Angles (rad) : Inport
  Demux : Demux  Outputs=3
  Demux1 : Demux  Outputs=3
  Gain : Gain  Gain=0.5
  Mux2 : Mux
  Product{,1..7} (8 alike) : Product  Inputs=***  RndMeth=Zero
  Reshape : Reshape  OutputDimensionality=Customize  OutputDimensions=[4,1]
  Sum : Sum  Inputs=|++
  Sum1 : Sum  Inputs=|+-
  Sum2 : Sum  Inputs=|++
  Sum3 : Sum  Inputs=|+-
  Trigonometric Function : Trigonometry
  Trigonometric Function1 : Trigonometry  Operator=cos
  Quat : Outport
  wires:
  Reshape/1 -> Quat/1
  Product7/1 -> Sum3/1
  Product6/1 -> Sum3/2
  Product2/1 -> Sum1/2
  Product3/1 -> Sum1/1
  Mux2/1 -> Reshape/1
  Sum3/1 -> Mux2/4
  Sum2/1 -> Mux2/3
  Product5/1 -> Sum2/2
  Product4/1 -> Sum2/1
  Sum1/1 -> Mux2/2
  Demux1/3 -> Product6/3, Product4/3, Product3/2, Product1/3
  Demux1/2 -> Product7/3, Product5/3, Product3/1, Product1/2
  Demux1/1 -> Product7/2, Product4/2, Product2/3, Product1/1
  Product1/1 -> Sum/2
  Demux/3 -> Product7/1, Product5/2, Product2/2, Product/3
  Demux/2 -> Product6/2, Product4/1, Product2/1, Product/2
  Demux/1 -> Product6/1, Product5/1, Product3/3, Product/1
  Product/1 -> Sum/1
  Euler Angles (rad)/1 -> Gain/1
  Trigonometric Function1/1 -> Demux1/1
  Trigonometric Function/1 -> Demux/1
  Sum/1 -> Mux2/1
  Gain/1 -> Trigonometric Function1/1, Trigonometric Function/1

== system OpenFlightUtilLib/Transformations/Euler_2_DCM ==
  note: Convert Euler Angles to Direction Cosine Matrix
  Euler Angles (rad) : Inport
  DCM_321 : OpenFlightUtilLib/Transformations/DCM_321
  Demux : Demux  Outputs=3
  Gain : Gain  Gain=rad2deg
      settings: AttributesFormatString=<%<BlockType> = '%<Gain>'>
  Trans : Outport
  wires:
  DCM_321/1 -> Trans/1
  Euler Angles (rad)/1 -> Gain/1
  Demux/1 -> DCM_321/1
  Demux/2 -> DCM_321/2
  Demux/3 -> DCM_321/3
  Gain/1 -> Demux/1

== system OpenFlightUtilLib/Transformations/Geodetic_2_TransE2L ==
  note: Geodetic to NED DCM
  "Pos Geodetic (deg, deg, m)" : Inport
  Constant1 : Constant  Value=90
  DCM_2_Rotation : OpenFlightUtilLib/Transformations/DCM_2_Rotation
  DCM_3_Rotation : OpenFlightUtilLib/Transformations/DCM_3_Rotation
  Demux2 : Demux  Outputs=3
  Gain1 : Gain  Gain=pi/180
      settings: AttributesFormatString=<%<BlockType> = '%<Gain>'>
  Gain2 : Gain  Gain=pi/180
      settings: AttributesFormatString=<%<BlockType> = '%<Gain>'>
  Gain3 : Gain  Gain=-1
  Product : Product  Multiplication=Matrix(*)  RndMeth=Zero
  Sum1 : Sum  Inputs=|++
  Terminator2 : Terminator
  Trans E2L : Outport
  wires:
  Gain1/1 -> DCM_2_Rotation/1
  Product/1 -> Trans E2L/1
  Demux2/1 -> Sum1/1
  Gain2/1 -> DCM_3_Rotation/1
  DCM_3_Rotation/1 -> Product/2
  DCM_2_Rotation/1 -> Product/1
  Demux2/3 -> Terminator2/1
  "Pos Geodetic (deg, deg, m)"/1 -> Demux2/1
  Demux2/2 -> Gain2/1
  Gain3/1 -> Gain1/1
  Sum1/1 -> Gain3/1
  Constant1/1 -> Sum1/2

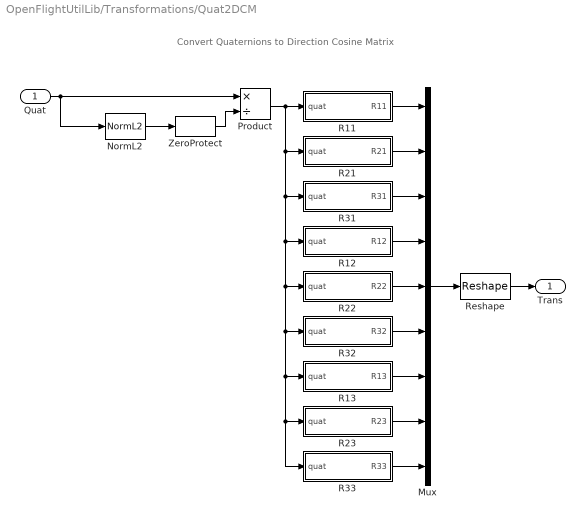
== system OpenFlightUtilLib/Transformations/Quat2DCM ==
  note: Convert Quaternions to Direction Cosine Matrix
  Quat : Inport
  Mux : Mux  Inputs=9
  NormL2 : OpenFlightUtilLib/Math/NormL2
  Product : Product  Inputs=*/
  R11 : Subsystem
  R12 : Subsystem
  R13 : Subsystem
  R21 : Subsystem
  R22 : Subsystem
  R23 : Subsystem
  R31 : Subsystem
  R32 : Subsystem
  R33 : Subsystem
  Reshape : Reshape  OutputDimensionality=Customize  OutputDimensions=[3, 3]
  ZeroProtect : OpenFlightUtilLib/Math/ZeroProtect  epsilon=eps
  Trans : Outport
  wires:
  NormL2/1 -> ZeroProtect/1
  R33/1(R33) -> Mux/9
  R23/1(R23) -> Mux/8
  R13/1(R13) -> Mux/7
  R32/1(R32) -> Mux/6
  R22/1(R22) -> Mux/5
  R12/1(R12) -> Mux/4
  R31/1(R31) -> Mux/3
  R21/1(R21) -> Mux/2
  R11/1(R11) -> Mux/1
  Mux/1 -> Reshape/1
  Product/1 -> R33/1(quat), R23/1(quat), R13/1(quat), R32/1(quat), R22/1(quat), R12/1(quat), R31/1(quat), R21/1(quat), R11/1(quat)
  ZeroProtect/1 -> Product/2
  Quat/1 -> NormL2/1, Product/1
  Reshape/1 -> Trans/1

== system OpenFlightUtilLib/Transformations/Quat2Euler ==
  note: Convert Quaternions to Euler Angles
  Quat : Inport
  Attitude : Subsystem
  Bank : Subsystem
  Heading : Subsystem
  L2Norm : OpenFlightUtilLib/Math/NormL2
  Mux1 : Mux  Inputs=3
  Product : Product  Inputs=*/
  Reshape : Reshape  OutputDimensionality=Customize  OutputDimensions=[3,1]
  ZeroProtect : OpenFlightUtilLib/Math/ZeroProtect  epsilon=eps
  Euler Angles (rad) : Outport
  wires:
  L2Norm/1 -> ZeroProtect/1
  ZeroProtect/1 -> Product/2
  Quat/1 -> L2Norm/1, Product/1
  Reshape/1 -> Euler Angles (rad)/1
  Heading/1(Heading Angle (rad)) -> Mux1/3
  Attitude/1(attitude angle (rad)) -> Mux1/2
  Product/1 -> Heading/1(Quat), Attitude/1(Quat), Bank/1(Quat)
  Bank/1(Bank Angle (rad)) -> Mux1/1
  Mux1/1 -> Reshape/1

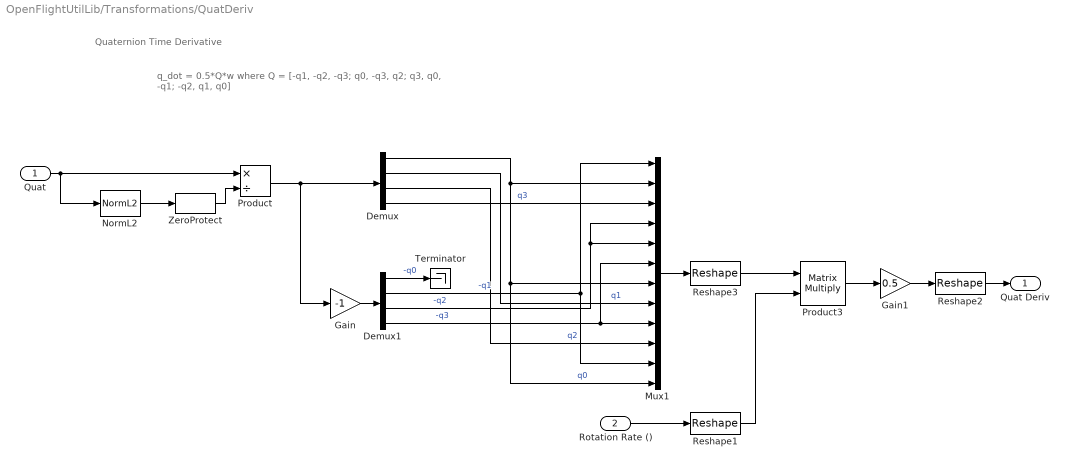
== system OpenFlightUtilLib/Transformations/QuatDeriv ==
  note: Quaternion Time Derivative
  note: q_dot = 0.5*Q*w
      | where Q = [-q1, -q2, -q3; q0, -q3, q2; q3, q0, -q1; -q2, q1, q0]
  Quat : Inport
  Rotation Rate () : Inport  Port=2
  Demux : Demux
  Demux1 : Demux
  Gain : Gain  Gain=-1
  Gain1 : Gain  Gain=0.5
  Mux1 : Mux  Inputs=12
  NormL2 : OpenFlightUtilLib/Math/NormL2
  Product : Product  Inputs=*/
  Product3 : Product  Multiplication=Matrix(*)  SaturateOnIntegerOverflow=on  OutDataTypeStr=Inherit: Same as first input
  Reshape1 : Reshape  OutputDimensionality=Customize  OutputDimensions=[3, 1]
  Reshape2 : Reshape  OutputDimensionality=Customize  OutputDimensions=[4, 1]
  Reshape3 : Reshape  OutputDimensionality=Customize  OutputDimensions=[4,3]
  Terminator : Terminator
  ZeroProtect : OpenFlightUtilLib/Math/ZeroProtect  epsilon=eps
  Quat Deriv : Outport
  wires:
  NormL2/1 -> ZeroProtect/1
  ZeroProtect/1 -> Product/2
  Quat/1 -> NormL2/1, Product/1
  Reshape2/1 -> Quat Deriv/1
  Product/1 -> Gain/1, Demux/1
  Reshape1/1 -> Product3/2
  Product3/1 -> Gain1/1
  Reshape3/1 -> Product3/1
  Gain1/1 -> Reshape2/1
  Demux1/1 -> Terminator/1  "-q0"
  Gain/1 -> Demux1/1
  Demux1/4 -> Mux1/9, Mux1/6  "-q3"
  Demux1/3 -> Mux1/5, Mux1/4  "-q2"
  Demux1/2 -> Mux1/11, Mux1/1  "-q1"
  Mux1/1 -> Reshape3/1
  Demux/4 -> Mux1/3  "q3"
  Demux/3 -> Mux1/10  "q2"
  Demux/2 -> Mux1/8  "q1"
  Demux/1 -> Mux1/12, Mux1/7, Mux1/2  "q0"
  Rotation Rate ()/1 -> Reshape1/1

== system OpenFlightUtilLib/Transformations/QuatInt ==
  note: Quaternion Integration
  Quat Rate : Inport
  Quat Init : Inport  Port=2
  Integrator : Integrator  InitialConditionSource=external  ContinuousStateAttributes='quatState'
      settings: AttributesFormatString=State: %<ContinuousStateAttributes>
  Reshape1 : Reshape  OutputDimensionality=Customize  OutputDimensions=[4,1]
  Reshape2 : Reshape  OutputDimensionality=Customize  OutputDimensions=[4,1]
  Reshape3 : Reshape  OutputDimensionality=Customize  OutputDimensions=[4,1]
  Quat : Outport
  wires:
  Reshape2/1 -> Quat/1
  Quat Init/1 -> Reshape1/1
  Reshape1/1 -> Integrator/2
  Reshape3/1 -> Integrator/1
  Quat Rate/1 -> Reshape3/1
  Integrator/1 -> Reshape2/1

== system OpenFlightUtilLib/Transformations/Quat2DCM/R11 ==
  quat : Inport
  Demux : Demux
  Math Function{,1..3} (4 alike) : Math  Operator=square  SaturateOnIntegerOverflow=on
  Sum1 : Sum  Inputs=++--
  R11 : Outport
  wires:
  Sum1/1 -> R11/1
  quat/1 -> Demux/1
  Math Function/1 -> Sum1/1
  Math Function1/1 -> Sum1/2
  Math Function2/1 -> Sum1/3
  Math Function3/1 -> Sum1/4
  Demux/1 -> Math Function/1
  Demux/2 -> Math Function1/1
  Demux/3 -> Math Function2/1
  Demux/4 -> Math Function3/1

== system OpenFlightUtilLib/Transformations/Quat2DCM/R12 ==
  quat : Inport
  Demux : Demux
  Gain : Gain  Gain=2
  Product1 : Product  Inputs=**
  Product2 : Product  Inputs=**
  Sum : Sum
  R12 : Outport
  wires:
  Demux/3 -> Product2/2
  Demux/2 -> Product2/1
  Demux/4 -> Product1/2
  Demux/1 -> Product1/1
  Sum/1 -> Gain/1
  Product2/1 -> Sum/2
  Product1/1 -> Sum/1
  quat/1 -> Demux/1
  Gain/1 -> R12/1

== system OpenFlightUtilLib/Transformations/Quat2DCM/R13 ==
  quat : Inport
  Demux : Demux
  Gain : Gain  Gain=2
  Product1 : Product  Inputs=**
  Product2 : Product  Inputs=**
  Sum : Sum  Inputs=+-
  R13 : Outport
  wires:
  Demux/4 -> Product1/2
  Demux/2 -> Product1/1
  Demux/3 -> Product2/2
  Demux/1 -> Product2/1
  Gain/1 -> R13/1
  quat/1 -> Demux/1
  Product1/1 -> Sum/1
  Product2/1 -> Sum/2
  Sum/1 -> Gain/1

== system OpenFlightUtilLib/Transformations/Quat2DCM/R21 ==
  quat : Inport
  Demux : Demux
  Gain : Gain  Gain=2
  Product1 : Product  Inputs=**
  Product2 : Product  Inputs=**
  Sum : Sum  Inputs=+-
  R21 : Outport
  wires:
  Demux/3 -> Product1/2
  Demux/2 -> Product1/1
  Demux/4 -> Product2/2
  Demux/1 -> Product2/1
  Sum/1 -> Gain/1
  Product2/1 -> Sum/2
  Product1/1 -> Sum/1
  quat/1 -> Demux/1
  Gain/1 -> R21/1

== system OpenFlightUtilLib/Transformations/Quat2DCM/R22 ==
  quat : Inport
  Demux : Demux
  Math Function{,1..3} (4 alike) : Math  Operator=square  SaturateOnIntegerOverflow=on
  Sum1 : Sum  Inputs=+-+-
  R22 : Outport
  wires:
  Demux/4 -> Math Function3/1
  Demux/3 -> Math Function2/1
  Demux/2 -> Math Function1/1
  Demux/1 -> Math Function/1
  Math Function3/1 -> Sum1/4
  Math Function2/1 -> Sum1/3
  Math Function1/1 -> Sum1/2
  Math Function/1 -> Sum1/1
  quat/1 -> Demux/1
  Sum1/1 -> R22/1

== system OpenFlightUtilLib/Transformations/Quat2DCM/R23 ==
  quat : Inport
  Demux : Demux
  Gain : Gain  Gain=2
  Product1 : Product  Inputs=**
  Product2 : Product  Inputs=**
  Sum : Sum
  R23 : Outport
  wires:
  Gain/1 -> R23/1
  quat/1 -> Demux/1
  Product1/1 -> Sum/1
  Product2/1 -> Sum/2
  Sum/1 -> Gain/1
  Demux/1 -> Product1/1
  Demux/2 -> Product1/2
  Demux/3 -> Product2/1
  Demux/4 -> Product2/2

== system OpenFlightUtilLib/Transformations/Quat2DCM/R31 ==
  quat : Inport
  Demux : Demux
  Gain : Gain  Gain=2
  Product1 : Product  Inputs=**
  Product2 : Product  Inputs=**
  Sum : Sum
  R31 : Outport
  wires:
  Demux/2 -> Product2/1
  Demux/3 -> Product1/2
  Demux/4 -> Product2/2
  Demux/1 -> Product1/1
  Sum/1 -> Gain/1
  Product2/1 -> Sum/2
  Product1/1 -> Sum/1
  quat/1 -> Demux/1
  Gain/1 -> R31/1

== system OpenFlightUtilLib/Transformations/Quat2DCM/R32 ==
  quat : Inport
  Demux : Demux
  Gain : Gain  Gain=2
  Product1 : Product  Inputs=**
  Product2 : Product  Inputs=**
  Sum : Sum  Inputs=+-
  R32 : Outport
  wires:
  Demux/4 -> Product1/2
  Demux/3 -> Product1/1
  Demux/2 -> Product2/2
  Demux/1 -> Product2/1
  Gain/1 -> R32/1
  quat/1 -> Demux/1
  Product1/1 -> Sum/1
  Product2/1 -> Sum/2
  Sum/1 -> Gain/1

== system OpenFlightUtilLib/Transformations/Quat2DCM/R33 ==
  quat : Inport
  Demux : Demux
  Math Function{,1..3} (4 alike) : Math  Operator=square  SaturateOnIntegerOverflow=on
  Sum1 : Sum  Inputs=+--+
  R33 : Outport
  wires:
  Sum1/1 -> R33/1
  quat/1 -> Demux/1
  Math Function/1 -> Sum1/1
  Math Function1/1 -> Sum1/2
  Math Function2/1 -> Sum1/3
  Math Function3/1 -> Sum1/4
  Demux/1 -> Math Function/1
  Demux/2 -> Math Function1/1
  Demux/3 -> Math Function2/1
  Demux/4 -> Math Function3/1

== system OpenFlightUtilLib/Transformations/Quat2Euler/Attitude ==
  Quat : Inport
  Demux : Demux
  Gain : Gain  Gain=2
  Product1 : Product  Inputs=**
  Product2 : Product  Inputs=**
  Sum : Sum  Inputs=+-
  Trigonometric Function : Trigonometry  Operator=asin
  attitude angle (rad) : Outport
  wires:
  Demux/4 -> Product2/2
  Demux/2 -> Product2/1
  Demux/3 -> Product1/2
  Demux/1 -> Product1/1
  Product1/1 -> Sum/1
  Product2/1 -> Sum/2
  Trigonometric Function/1 -> attitude angle (rad)/1
  Quat/1 -> Demux/1
  Sum/1 -> Gain/1
  Gain/1 -> Trigonometric Function/1

== system OpenFlightUtilLib/Transformations/Quat2Euler/Bank ==
  Quat : Inport
  Demux : Demux
  Gain : Gain  Gain=2
  Math Function{,1..3} (4 alike) : Math  Operator=square  SaturateOnIntegerOverflow=on
  Product1 : Product  Inputs=**
  Product2 : Product  Inputs=**
  Sum : Sum
  Sum1 : Sum  Inputs=+--+
  Trigonometric Function : Trigonometry  Operator=atan2
  Bank Angle (rad) : Outport
  wires:
  Demux/4 -> Product2/2, Math Function3/1
  Demux/3 -> Product2/1, Math Function2/1
  Demux/2 -> Product1/2, Math Function1/1
  Demux/1 -> Product1/1, Math Function/1
  Sum1/1 -> Trigonometric Function/2
  Math Function3/1 -> Sum1/4
  Math Function2/1 -> Sum1/3
  Math Function1/1 -> Sum1/2
  Math Function/1 -> Sum1/1
  Gain/1 -> Trigonometric Function/1
  Sum/1 -> Gain/1
  Product2/1 -> Sum/2
  Product1/1 -> Sum/1
  Quat/1 -> Demux/1
  Trigonometric Function/1 -> Bank Angle (rad)/1

== system OpenFlightUtilLib/Transformations/Quat2Euler/Heading ==
  Quat : Inport
  Demux : Demux
  Gain : Gain  Gain=2
  Math Function{,1..3} (4 alike) : Math  Operator=square  SaturateOnIntegerOverflow=on
  Product1 : Product  Inputs=**
  Product2 : Product  Inputs=**
  Sum : Sum
  Sum1 : Sum  Inputs=++--
  Trigonometric Function : Trigonometry  Operator=atan2
  Heading Angle (rad) : Outport
  wires:
  Demux/4 -> Product1/2, Math Function3/1
  Demux/3 -> Product2/2, Math Function2/1
  Demux/2 -> Product2/1, Math Function1/1
  Demux/1 -> Product1/1, Math Function/1
  Sum1/1 -> Trigonometric Function/2
  Math Function3/1 -> Sum1/4
  Math Function2/1 -> Sum1/3
  Math Function1/1 -> Sum1/2
  Math Function/1 -> Sum1/1
  Gain/1 -> Trigonometric Function/1
  Sum/1 -> Gain/1
  Product2/1 -> Sum/2
  Product1/1 -> Sum/1
  Quat/1 -> Demux/1
  Trigonometric Function/1 -> Heading Angle (rad)/1
